simulink model "Exercicio_1g_sim"  (R2016a)
settings: Solver=VariableStepAuto  StartTime=0.0  StopTime=t_sim  RelTol=1e-3
values from neighbouring files (symbols this model uses):
  A_AObs = (A_Abb-(A_Ke*A_Aab))    [Exercicio_1.m]    (also in Exercicio_1_teste.m)
  A_BObs = ((A_AObs*A_Ke) + A_Aba - (A_Ke*A_Aaa))    [Exercicio_1.m]    (also in Exercicio_1_teste.m = ((A_AObs*Ke) + A_Aba - (A_Ke*A_Aaa)))
  A_CObs = [[0 0];[eye(2)]]    [Exercicio_1.m]    (also in Exercicio_1_teste.m = (eye(2)))
  A_DObs = [1;A_Ke]    [Exercicio_1.m]    (also in Exercicio_1_teste.m)
  A_FObs = (A_Bb - (A_Ke*A_Ba))    [Exercicio_1.m]    (also in Exercicio_1_teste.m)
  A_K_cntrl = acker(A,B, p_mf)    [Exercicio_1.m]
undefined symbols (not defined in the file or in its folder): A_susp, Aa_susp, B_susp, Ba_susp, C_susp, Ca_susp, D_susp, Da_susp, K_susp, Keobs_susp
settings Model: Creator=Usuario  LastModifiedBy=Eletrônica Auto Poli

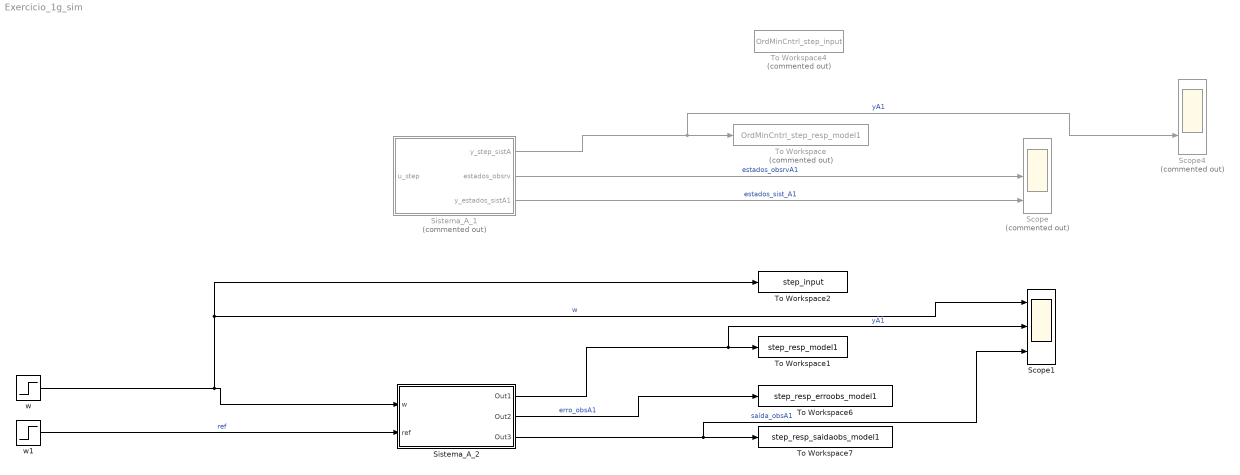
== system Exercicio_1g_sim ==
  Scope : Scope  Commented=on  NumInputPorts=3
  Scope1 : Scope  NumInputPorts=3
  Scope4 : Scope  Commented=on  NumInputPorts=2
  Sistema_A_1 : Subsystem  Commented=on
  Sistema_A_2 : Subsystem
  To Workspace : ToWorkspace  Commented=on  VariableName=OrdMinCntrl_step_resp_model1  SaveFormat=Timeseries  SampleTime=-1
  To Workspace1 : ToWorkspace  VariableName=step_resp_model1  SaveFormat=Timeseries  SampleTime=-1
  To Workspace2 : ToWorkspace  VariableName=step_input  SaveFormat=Timeseries  SampleTime=-1
  To Workspace4 : ToWorkspace  Commented=on  VariableName=OrdMinCntrl_step_input  SaveFormat=Timeseries  SampleTime=-1
  To Workspace6 : ToWorkspace  VariableName=step_resp_erroobs_model1  SaveFormat=Timeseries  SampleTime=-1
  To Workspace7 : ToWorkspace  VariableName=step_resp_saidaobs_model1  SaveFormat=Timeseries  SampleTime=-1
  w : Step  After=0  SampleTime=0.01
  w1 : Step  SampleTime=0.01
  wires:
  Sistema_A_1/1(y_step_sistA) -> Scope4/2, To Workspace/1  "yA1"
  Sistema_A_1/2(estados_obsrv) -> Scope/2  "estados_obsrvA1"
  Sistema_A_1/3(y_estados_sistA1) -> Scope/3  "estados_sist_A1"
  Sistema_A_2/1(Out1) -> Scope1/2, To Workspace1/1  "yA1"
  Sistema_A_2/2(Out2) -> To Workspace6/1  "erro_obsA1"
  Sistema_A_2/3(Out3) -> Scope1/3, To Workspace7/1  "saída_obsA1"
  w/1 -> Scope1/1, To Workspace2/1, Sistema_A_2/1(w)  "w"
  w1/1 -> Sistema_A_2/2(ref)  "ref"

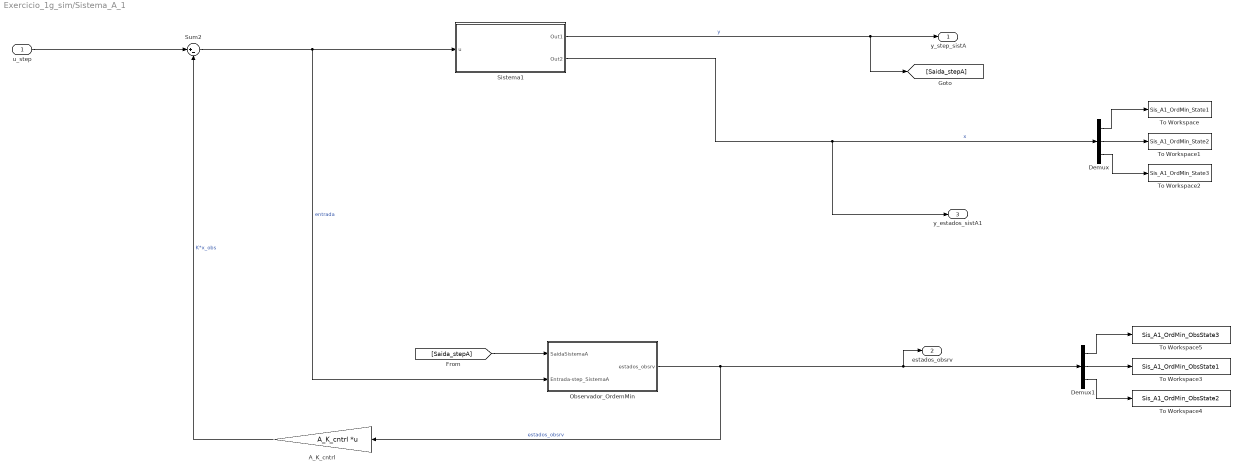
== system Exercicio_1g_sim/Sistema_A_1 ==
  u_step : Inport
  A_K_cntrl : Gain  Gain=A_K_cntrl  Multiplication=Matrix(K*u)
  Demux : Demux  Outputs=3
  Demux1 : Demux  Outputs=3
  Observador_OrdemMin : Subsystem
  Sistema1 : Subsystem
  Sum2 : Sum  Inputs=|+-
  To Workspace : ToWorkspace  VariableName=Sis_A1_OrdMin_State1  SaveFormat=Timeseries  SampleTime=-1
  To Workspace1 : ToWorkspace  VariableName=Sis_A1_OrdMin_State2  SaveFormat=Timeseries  SampleTime=-1
  To Workspace2 : ToWorkspace  VariableName=Sis_A1_OrdMin_State3  SaveFormat=Timeseries  SampleTime=-1
  To Workspace3 : ToWorkspace  VariableName=Sis_A1_OrdMin_ObsState1  SaveFormat=Timeseries  SampleTime=-1
  To Workspace4 : ToWorkspace  VariableName=Sis_A1_OrdMin_ObsState2  SaveFormat=Timeseries  SampleTime=-1
  To Workspace5 : ToWorkspace  VariableName=Sis_A1_OrdMin_ObsState3  SaveFormat=Timeseries  SampleTime=-1
  y_step_sistA : Outport
  estados_obsrv : Outport  Port=2
  y_estados_sistA1 : Outport  Port=3
  wires:
  Demux/1 -> To Workspace/1
  Demux/2 -> To Workspace1/1
  Demux/3 -> To Workspace2/1
  Sum2/1 -> Sistema1/1(u), Observador_OrdemMin/2(Entrada-step_SistemaA)  "entrada"
  Sistema1/1(Out1) -> [Saida_stepA], y_step_sistA/1  "y"
  Sistema1/2(Out2) -> y_estados_sistA1/1, Demux/1  "x"
  Demux1/1 -> To Workspace5/1
  Demux1/2 -> To Workspace3/1
  Demux1/3 -> To Workspace4/1
  Observador_OrdemMin/1(estados_obsrv) -> A_K_cntrl/1, estados_obsrv/1, Demux1/1  "estados_obsrv"
  [Saida_stepA] -> Observador_OrdemMin/1(SaidaSistemaA)
  A_K_cntrl/1 -> Sum2/2  "K*x_obs"
  u_step/1 -> Sum2/1

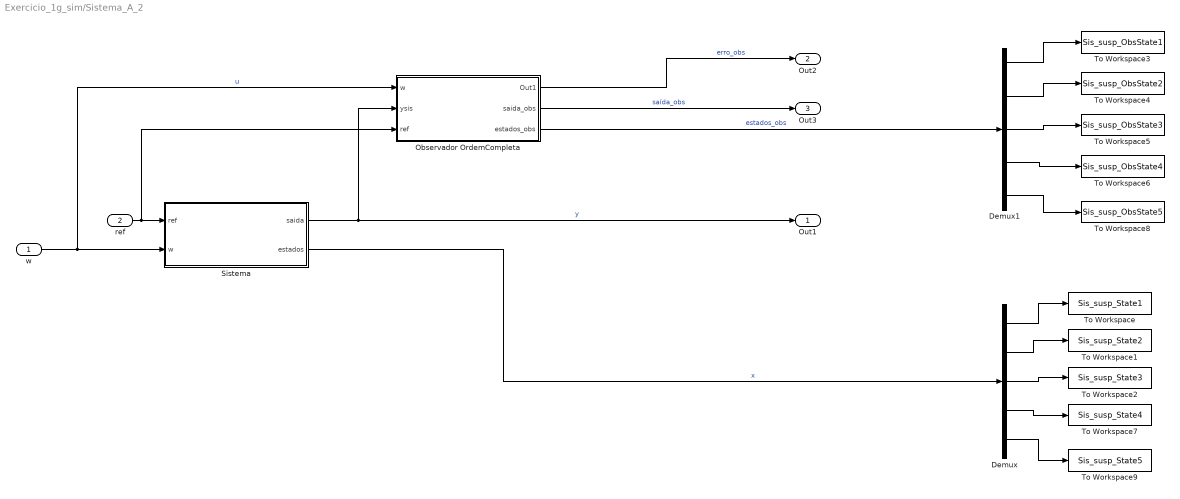
== system Exercicio_1g_sim/Sistema_A_2 ==
  w : Inport
  ref : Inport  Port=2
  Demux : Demux  Outputs=5
  Demux1 : Demux  Outputs=5
  Observador OrdemCompleta : Subsystem
  Sistema : Subsystem
  To Workspace : ToWorkspace  VariableName=Sis_susp_State1  SaveFormat=Timeseries  SampleTime=-1
  To Workspace1 : ToWorkspace  VariableName=Sis_susp_State2  SaveFormat=Timeseries  SampleTime=-1
  To Workspace2 : ToWorkspace  VariableName=Sis_susp_State3  SaveFormat=Timeseries  SampleTime=-1
  To Workspace3 : ToWorkspace  VariableName=Sis_susp_ObsState1  SaveFormat=Timeseries  SampleTime=-1
  To Workspace4 : ToWorkspace  VariableName=Sis_susp_ObsState2  SaveFormat=Timeseries  SampleTime=-1
  To Workspace5 : ToWorkspace  VariableName=Sis_susp_ObsState3  SaveFormat=Timeseries  SampleTime=-1
  To Workspace6 : ToWorkspace  VariableName=Sis_susp_ObsState4  SaveFormat=Timeseries  SampleTime=-1
  To Workspace7 : ToWorkspace  VariableName=Sis_susp_State4  SaveFormat=Timeseries  SampleTime=-1
  To Workspace8 : ToWorkspace  VariableName=Sis_susp_ObsState5  SaveFormat=Timeseries  SampleTime=-1
  To Workspace9 : ToWorkspace  VariableName=Sis_susp_State5  SaveFormat=Timeseries  SampleTime=-1
  Out1 : Outport
  Out2 : Outport  Port=2
  Out3 : Outport  Port=3
  wires:
  Demux/1 -> To Workspace/1
  Demux/2 -> To Workspace1/1
  Demux/3 -> To Workspace2/1
  Sistema/1(saida) -> Out1/1, Observador OrdemCompleta/2(ysis)  "y"
  Sistema/2(estados) -> Demux/1  "x"
  Demux1/1 -> To Workspace3/1
  Demux1/2 -> To Workspace4/1
  Demux1/3 -> To Workspace5/1
  Observador OrdemCompleta/1(Out1) -> Out2/1  "erro_obs"
  Observador OrdemCompleta/2(saida_obs) -> Out3/1  "saída_obs"
  Observador OrdemCompleta/3(estados_obs) -> Demux1/1  "estados_obs"
  Demux1/4 -> To Workspace6/1
  Demux/4 -> To Workspace7/1
  Demux1/5 -> To Workspace8/1
  Demux/5 -> To Workspace9/1
  w/1 -> Sistema/2(w), Observador OrdemCompleta/1(w)  "u"
  ref/1 -> Sistema/1(ref), Observador OrdemCompleta/3(ref)

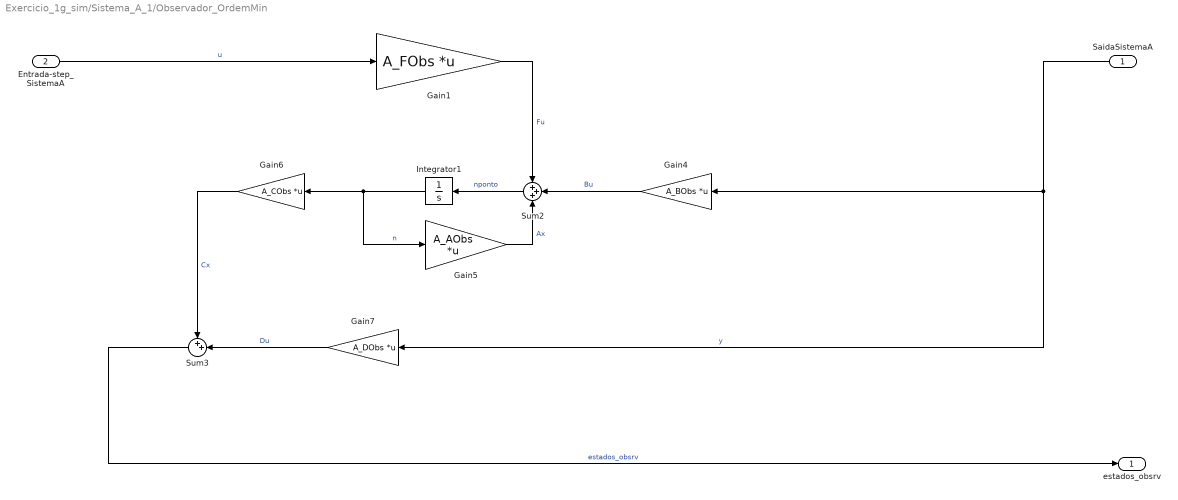
== system Exercicio_1g_sim/Sistema_A_1/Observador_OrdemMin ==
  SaidaSistemaA : Inport
  Entrada-step_SistemaA : Inport  Port=2
  Gain1 : Gain  Gain=A_FObs  Multiplication=Matrix(K*u)
  Gain4 : Gain  Gain=A_BObs  Multiplication=Matrix(K*u)
  Gain5 : Gain  Gain=A_AObs  Multiplication=Matrix(K*u)
  Gain6 : Gain  Gain=A_CObs  Multiplication=Matrix(K*u)
  Gain7 : Gain  Gain=A_DObs  Multiplication=Matrix(K*u)
  Integrator1 : Integrator  UpperSaturationLimit=1.279387983436996e+55  LowerSaturationLimit=0
  Sum2 : Sum  Inputs=+++
  Sum3 : Sum  Inputs=++|
  estados_obsrv : Outport
  wires:
  Integrator1/1 -> Gain5/1, Gain6/1  "n"
  Gain6/1 -> Sum3/1  "Cx"
  SaidaSistemaA/1 -> Gain4/1, Gain7/1  "y"
  Sum3/1 -> estados_obsrv/1  "estados_obsrv"
  Gain7/1 -> Sum3/2  "Du"
  Gain4/1 -> Sum2/2  "Bu"
  Gain5/1 -> Sum2/3  "Ax"
  Gain1/1 -> Sum2/1  "Fu"
  Sum2/1 -> Integrator1/1  "nponto"
  Entrada-step_SistemaA/1 -> Gain1/1  "u"

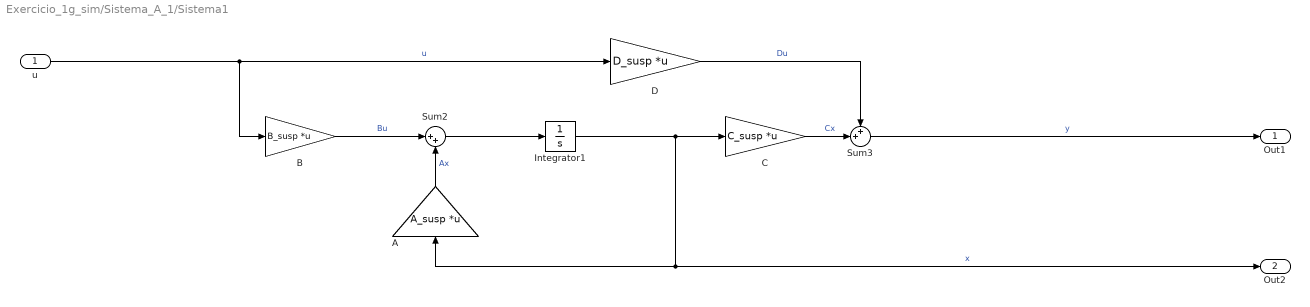
== system Exercicio_1g_sim/Sistema_A_1/Sistema1 ==
  u : Inport
  A : Gain  Gain=A_susp  Multiplication=Matrix(K*u)
  B : Gain  Gain=B_susp  Multiplication=Matrix(K*u)
  C : Gain  Gain=C_susp  Multiplication=Matrix(K*u)
  D : Gain  Gain=D_susp  Multiplication=Matrix(K*u)
  Integrator1 : Integrator
  Sum2 : Sum  Inputs=|++
  Sum3 : Sum  Inputs=++|
  Out1 : Outport
  Out2 : Outport  Port=2
  wires:
  u/1 -> B/1, D/1  "u"
  Sum3/1 -> Out1/1  "y"
  Integrator1/1 -> A/1, Out2/1, C/1  "x"
  C/1 -> Sum3/2  "Cx"
  D/1 -> Sum3/1  "Du"
  B/1 -> Sum2/1  "Bu"
  A/1 -> Sum2/2  "Ax"
  Sum2/1 -> Integrator1/1

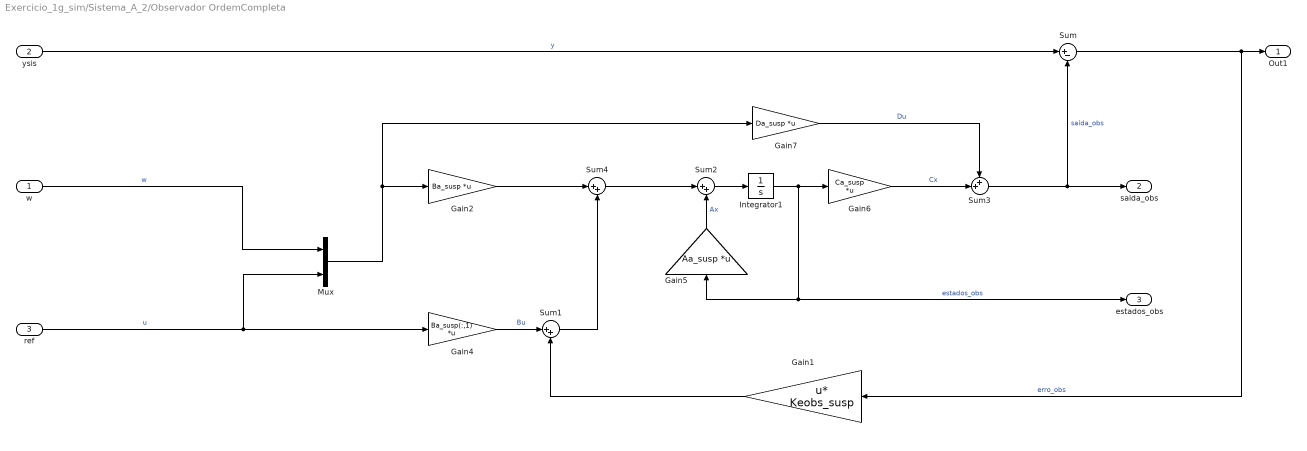
== system Exercicio_1g_sim/Sistema_A_2/Observador OrdemCompleta ==
  w : Inport
  ysis : Inport  Port=2
  ref : Inport  Port=3
  Gain1 : Gain  Gain=Keobs_susp  Multiplication=Matrix(u*K)
  Gain2 : Gain  Gain=Ba_susp  Multiplication=Matrix(K*u)
  Gain4 : Gain  Gain=Ba_susp(:,1)  Multiplication=Matrix(K*u)
  Gain5 : Gain  Gain=Aa_susp  Multiplication=Matrix(K*u)
  Gain6 : Gain  Gain=Ca_susp  Multiplication=Matrix(K*u)
  Gain7 : Gain  Gain=Da_susp  Multiplication=Matrix(K*u)
  Integrator1 : Integrator
  Mux : Mux  Inputs=2
  Sum : Sum  Inputs=|+-
  Sum1 : Sum  Inputs=|++
  Sum2 : Sum  Inputs=|++
  Sum3 : Sum  Inputs=++|
  Sum4 : Sum  Inputs=|++
  Out1 : Outport
  saida_obs : Outport  Port=2
  estados_obs : Outport  Port=3
  wires:
  Sum3/1 -> saida_obs/1, Sum/2  "saída_obs"
  Integrator1/1 -> estados_obs/1, Gain5/1, Gain6/1  "estados_obs"
  Gain6/1 -> Sum3/2  "Cx"
  Gain7/1 -> Sum3/1  "Du"
  Gain4/1 -> Sum1/1  "Bu"
  Gain5/1 -> Sum2/2  "Ax"
  Sum2/1 -> Integrator1/1
  ysis/1 -> Sum/1  "y"
  Sum/1 -> Out1/1, Gain1/1  "erro_obs"
  Sum1/1 -> Sum4/2
  Gain1/1 -> Sum1/2
  ref/1 -> Gain4/1, Mux/2  "u"
  w/1 -> Mux/1  "w"
  Sum4/1 -> Sum2/1
  Gain2/1 -> Sum4/1
  Mux/1 -> Gain7/1, Gain2/1

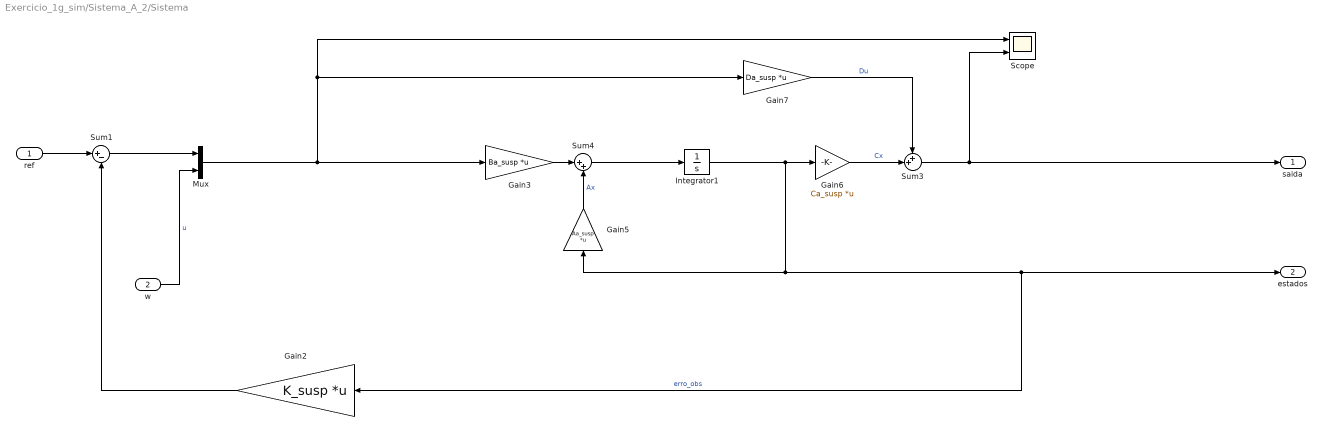
== system Exercicio_1g_sim/Sistema_A_2/Sistema ==
  ref : Inport
  w : Inport  Port=2
  Gain2 : Gain  Gain=K_susp  Multiplication=Matrix(K*u)
  Gain3 : Gain  Gain=Ba_susp  Multiplication=Matrix(K*u)
  Gain5 : Gain  Gain=Aa_susp  Multiplication=Matrix(K*u)
  Gain6 : Gain  Gain=Ca_susp  Multiplication=Matrix(K*u)
  Gain7 : Gain  Gain=Da_susp  Multiplication=Matrix(K*u)
  Integrator1 : Integrator  InitialCondition=[0 0 0 0 0]
  Mux : Mux  Inputs=2
  Scope : Scope  NumInputPorts=2
  Sum1 : Sum  Inputs=|+-
  Sum3 : Sum  Inputs=++|
  Sum4 : Sum  Inputs=|++
  saida : Outport
  estados : Outport  Port=2
  wires:
  Gain6/1 -> Sum3/2  "Cx"
  Gain5/1 -> Sum4/2  "Ax"
  Sum4/1 -> Integrator1/1
  Integrator1/1 -> Gain2/1, estados/1, Gain5/1, Gain6/1  "erro_obs"
  Gain3/1 -> Sum4/1
  Gain7/1 -> Sum3/1  "Du"
  Sum3/1 -> Scope/2, saida/1
  Mux/1 -> Gain7/1, Scope/1, Gain3/1
  Gain2/1 -> Sum1/2
  w/1 -> Mux/2  "u"
  Sum1/1 -> Mux/1
  ref/1 -> Sum1/1
